simulink model "formation_trajectory_tracking"  (R2022a)
settings: Solver=FixedStepAuto  StartTime=0  StopTime=80  FixedStep=0.01  RelTol=1e-3
settings Model: NumberOfSteps=100  Creator=11536  LastModifiedBy=11536
settings SolverCC: AlgebraicLoopSolver=TrustRegion
settings DataIOCC: ReturnWorkspaceOutputs=off
settings DebuggingCC: ArithmeticOperatorsInVariantConditions=warning
settings SFSimCC: CustomCodeUndefinedFunction=UseInterfaceOnly
settings CodeAppCC: StateflowObjectComments=on

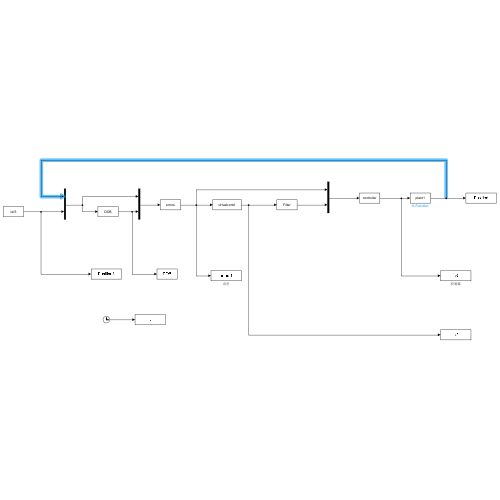
[thumbnail: Simulink's stored preview of the top-level diagram]
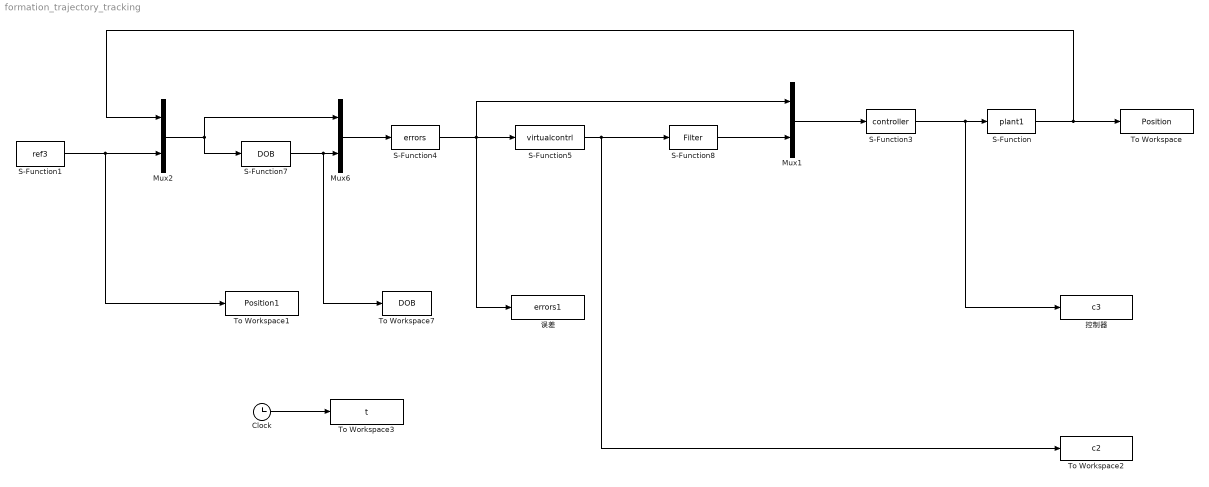
== system formation_trajectory_tracking ==
  Clock : Clock
  Mux1 : Mux  Inputs=2
  Mux2 : Mux  Inputs=2
  Mux6 : Mux  Inputs=2
  S-Function : S-Function  FunctionName=plant1  SFunctionDeploymentMode=off  EnableBusSupport=off
  S-Function1 : S-Function  FunctionName=ref3  SFunctionDeploymentMode=off  EnableBusSupport=off
  S-Function3 : S-Function  FunctionName=controller  SFunctionDeploymentMode=off  EnableBusSupport=off
  S-Function4 : S-Function  FunctionName=errors  SFunctionDeploymentMode=off  EnableBusSupport=off
  S-Function5 : S-Function  FunctionName=virtualcontrl  SFunctionDeploymentMode=off  EnableBusSupport=off
  S-Function7 : S-Function  FunctionName=DOB  SFunctionDeploymentMode=off  EnableBusSupport=off
  S-Function8 : S-Function  FunctionName=Filter  SFunctionDeploymentMode=off  EnableBusSupport=off
  To Workspace : ToWorkspace  VariableName=Position  SampleTime=-1
  To Workspace1 : ToWorkspace  VariableName=Position1  SampleTime=-1
  To Workspace2 : ToWorkspace  VariableName=c2  SampleTime=-1
  To Workspace3 : ToWorkspace  VariableName=t  SampleTime=-1
  To Workspace7 : ToWorkspace  VariableName=DOB  SampleTime=-1
  控制器 : ToWorkspace  VariableName=c3  SampleTime=-1
  误差 : ToWorkspace  VariableName=errors1  SampleTime=-1
  wires:
  Clock/1 -> To Workspace3/1
  Mux1/1 -> S-Function3/1
  S-Function3/1 -> 控制器/1, S-Function/1
  S-Function8/1 -> Mux1/2
  S-Function1/1 -> To Workspace1/1, Mux2/2
  Mux2/1 -> Mux6/1, S-Function7/1
  S-Function/1 -> To Workspace/1, Mux2/1
  S-Function5/1 -> To Workspace2/1, S-Function8/1
  Mux6/1 -> S-Function4/1
  S-Function7/1 -> To Workspace7/1, Mux6/2
  S-Function4/1 -> Mux1/1, 误差/1, S-Function5/1
